simulink model "Car_Control_A"  (R2023b)
settings: Solver=VariableStepAuto  StartTime=0.0  StopTime=300  RelTol=1e-3
libraries: fuzblock x1
settings Model: Creator=User  LastModifiedBy=user
settings DebuggingCC: UnconnectedInputMsg=warning  UnconnectedOutputMsg=warning  UnconnectedLineMsg=warning
settings ModelReferenceCC: EnableRefExpFcnMdlSchedulingChecks=on
settings RTWCC: DLArmComputeVersion=19.05

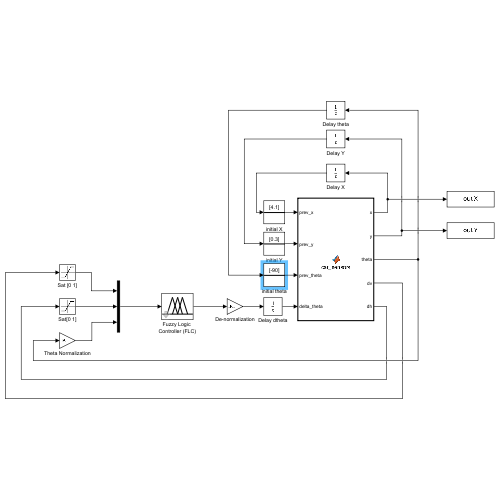
[thumbnail: Simulink's stored preview of the top-level diagram]
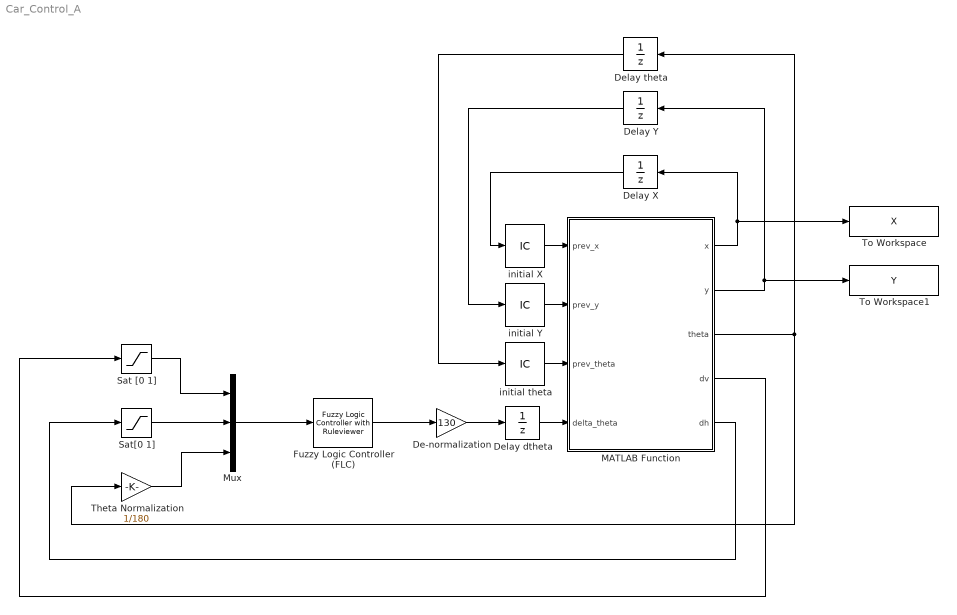
== system Car_Control_A ==
  De-normalization : Gain  Gain=130
  Delay X : UnitDelay  SampleTime=0.1  HasFrameUpgradeWarning=on
  Delay Y : UnitDelay  SampleTime=0.1  HasFrameUpgradeWarning=on
  Delay dtheta : UnitDelay  SampleTime=0.1  HasFrameUpgradeWarning=on
  Delay theta : UnitDelay  SampleTime=0.1  HasFrameUpgradeWarning=on
  Fuzzy Logic Controller (FLC) : fuzblock/Fuzzy Logic  Controller  with Ruleviewer  fismatrix=Car_Control_FIS_Tuned14  Ts=0.1
  MATLAB Function : MATLAB Function  TreatAsAtomicUnit=on
  Mux : Mux  Inputs=3
  Sat [0 1] : Saturate  UpperLimit=1  LowerLimit=0
  Sat[0 1] : Saturate  UpperLimit=1  LowerLimit=0
  Theta Normalization : Gain  Gain=1/180
  To Workspace : ToWorkspace  VariableName=X  SaveFormat=Timeseries  SampleTime=-1
  To Workspace1 : ToWorkspace  VariableName=Y  SaveFormat=Timeseries  SampleTime=-1
  initial X : InitialCondition  Value=4.1
  initial Y : InitialCondition  Value=0.3
  initial theta : InitialCondition  Value=-90
  wires:
  MATLAB Function/3(theta) -> Delay theta/1, Theta Normalization/1
  Delay theta/1 -> initial theta/1
  MATLAB Function/2(y) -> To Workspace1/1, Delay Y/1
  Delay Y/1 -> initial Y/1
  MATLAB Function/1(x) -> To Workspace/1, Delay X/1
  Delay X/1 -> initial X/1
  Fuzzy Logic Controller (FLC)/1 -> De-normalization/1
  De-normalization/1 -> Delay dtheta/1
  Mux/1 -> Fuzzy Logic Controller (FLC)/1
  MATLAB Function/4(dv) -> Sat [0 1]/1
  MATLAB Function/5(dh) -> Sat[0 1]/1
  Theta Normalization/1 -> Mux/3
  initial X/1 -> MATLAB Function/1(prev_x)
  initial Y/1 -> MATLAB Function/2(prev_y)
  initial theta/1 -> MATLAB Function/3(prev_theta)
  Sat[0 1]/1 -> Mux/2
  Sat [0 1]/1 -> Mux/1
  Delay dtheta/1 -> MATLAB Function/4(delta_theta)

== matlab function Car_Control_A/MATLAB Function ==
  data: x output; prev_x input; y output; prev_y input; prev_theta input; delta_theta input; theta output; dv output; dh output
% A function that represents the sensors of the car, setting the boundaries
% for any change on the car's route

function [x, y, theta, dv, dh] = car_sensors(prev_x, prev_y, prev_theta, delta_theta)
    
    if(prev_x >= 10)
        u = 0;
    else
        u = 0.05;       % Speed
    end
    
    t = 0.1;       % Delay between each calculation
    
    % Calculate the new angle of the car:
    theta = prev_theta + delta_theta;
    
    % Saturation for the new theta inside the [-180 180] 
    if(theta > 180)
        theta = 180;
    elseif(theta < -180)
       theta = -180;
    end
    
    % Calculation of the new position
    x = prev_x + u*cos(theta/360*2*pi)*t;
    y = prev_y + u*sin(theta/360*2*pi)*t;
    
    % Calculation of the horizontal distance from obstacle
    if (y <= 1)
        dh = 5 - x;
    elseif (y > 1 && y <= 2)
        dh = 6 - x;
    elseif (y > 2 && y <= 3)
        dh = 7 - x;
    else
        dh = 20 - x;
    end
    
    % Calculation of the vertical distance from obstacle
    if (x <= 5)
        dv = y;
    elseif (x > 5 && x <= 6)
        dv = y - 1;
    elseif (x > 6 && x <= 7)
        dv = y - 2;
    else
        dv = y - 3;
    end
end
